simulink model "avg_model"  (R2018a)
settings: Solver=ode4  StartTime=0.0  StopTime=Ttotal  FixedStep=Ts  RelTol=1e-3
values from neighbouring files (symbols this model uses):
  D = 2.0    (= 2)    [avg_model_script.m]
  Dmin = b / (rss * (1-rtr))    (= 1.90222222222)    [avg_model_script.m]
  M = 10.2    [avg_model_script.m]
  rtr = 0.1    [avg_model_script.m]
  Tstep = 0.5    [avg_model_script.m]
  x0 = 0    [avg_model_script.m]
undefined symbols (not defined in the file or in its folder): Pb
settings Model: Creator=ericfa  LastModifiedBy=ericfa

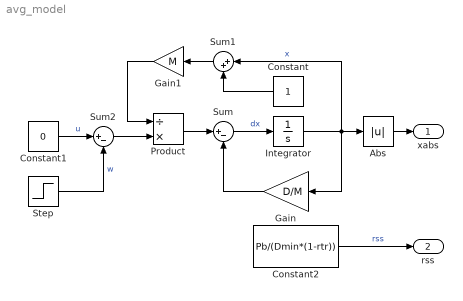
== system avg_model ==
  Abs : Abs
  Constant : Constant
  Constant1 : Constant  Value=0
  Constant2 : Constant  Value=Pb/(Dmin*(1-rtr))
  Gain : Gain  Gain=D/M
  Gain1 : Gain  Gain=M
  Integrator : Integrator  InitialCondition=x0
  Product : Product  Inputs=/*
  Step : Step  Time=Tstep  After=Pb  SampleTime=0
  Sum : Sum  Inputs=|+-
  Sum1 : Sum  Inputs=|++
  Sum2 : Sum  Inputs=|+-
  xabs : Outport
  rss : Outport  Port=2
  wires:
  Gain/1 -> Sum/2
  Sum/1 -> Integrator/1  "dx"
  Integrator/1 -> Abs/1, Gain/1, Sum1/1  "x"
  Product/1 -> Sum/1
  Sum1/1 -> Gain1/1
  Constant/1 -> Sum1/2
  Gain1/1 -> Product/1
  Sum2/1 -> Product/2
  Constant1/1 -> Sum2/1  "u"
  Step/1 -> Sum2/2  "w"
  Constant2/1 -> rss/1  "rss"
  Abs/1 -> xabs/1
